simulink model "resonance_pulse2a"  (R2022a)
settings: Solver=VariableStepAuto  StartTime=0.0  StopTime=223  MaxStep=1e-3  RelTol=1e-3
undefined symbols (not defined in the file): i
libraries: resonance_lib x2
settings Model: Creator=tstef  LastModifiedBy=tstef

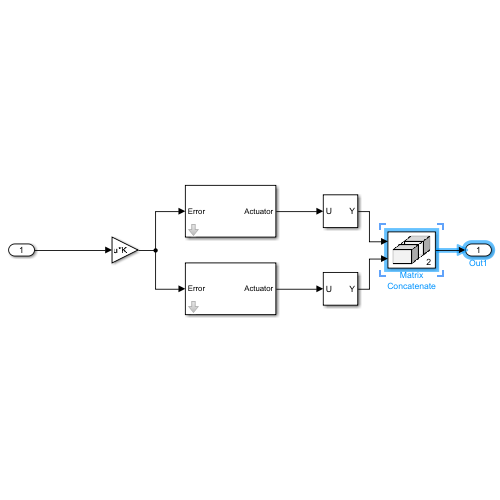
[thumbnail: Simulink's stored preview of the top-level diagram]
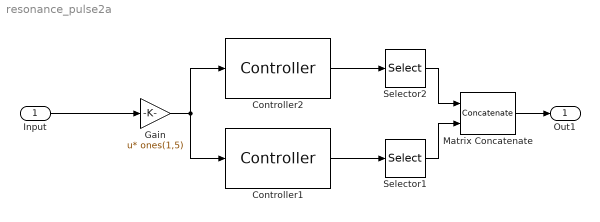
== system resonance_pulse2a ==
  Input : Inport
  Controller1 : resonance_lib/Controller  k_P=0  k_I=0  k_R=950+390*i  k_Rb=-3.9e5  T1=0.094  w0=100  zeta=0.05
  Controller2 : resonance_lib/Controller  k_P=43  k_I=10  k_R=0  k_Rb=0  T1=0.094  w0=100  zeta=0.05
  Gain : Gain  Gain=ones(1,5)  Multiplication=Matrix(u*K)
  Matrix Concatenate : Concatenate  Mode=Multidimensional array  ConcatenateDimension=2
  Selector1 : Selector  NumberOfDimensions=2  InputPortWidth=3  IndexOptions=Select all,Index vector (dialog)  Indices=[1 3],2  OutputSizes=1,1
  Selector2 : Selector  NumberOfDimensions=2  InputPortWidth=3  IndexOptions=Select all,Index vector (dialog)  Indices=[1 3],1  OutputSizes=1,1
  Out1 : Outport
  wires:
  Controller1/1 -> Selector1/1
  Selector1/1 -> Matrix Concatenate/2
  Input/1 -> Gain/1
  Gain/1 -> Controller1/1, Controller2/1
  Controller2/1 -> Selector2/1
  Selector2/1 -> Matrix Concatenate/1
  Matrix Concatenate/1 -> Out1/1
